simulink model "MUX_8BIT"  (R2018a)
settings: Solver=VariableStepAuto  StartTime=0.0  StopTime=10.0  RelTol=1e-3
settings Model: Creator=midog  LastModifiedBy=midog

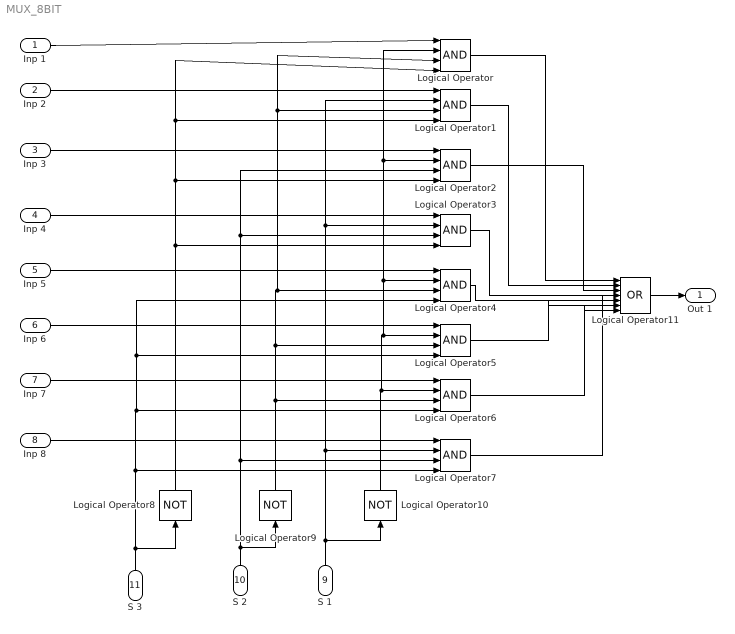
== system MUX_8BIT ==
  Inp 1 : Inport
  Inp 2 : Inport  Port=2
  Inp 3 : Inport  Port=3
  Inp 4 : Inport  Port=4
  Inp 5 : Inport  Port=5
  Inp 6 : Inport  Port=6
  Inp 7 : Inport  Port=7
  Inp 8 : Inport  Port=8
  S 1 : Inport  Port=9
  S 2 : Inport  Port=10
  S 3 : Inport  Port=11
  Logical Operator{,1..7} (8 alike) : Logic  Inputs=4  IconShape=distinctive  AllPortsSameDT=off  OutDataTypeStr=boolean
  Logical Operator10 : Logic  Operator=NOT  Inputs=4  IconShape=distinctive  AllPortsSameDT=off  OutDataTypeStr=boolean
  Logical Operator11 : Logic  Operator=OR  Inputs=8  IconShape=distinctive  AllPortsSameDT=off  OutDataTypeStr=boolean
  Logical Operator8 : Logic  Operator=NOT  Inputs=4  IconShape=distinctive  AllPortsSameDT=off  OutDataTypeStr=boolean
  Logical Operator9 : Logic  Operator=NOT  Inputs=4  IconShape=distinctive  AllPortsSameDT=off  OutDataTypeStr=boolean
  Out 1 : Outport
  wires:
  Inp 1/1 -> Logical Operator/1
  Inp 2/1 -> Logical Operator1/1
  Inp 3/1 -> Logical Operator2/1
  Inp 4/1 -> Logical Operator3/1
  Inp 5/1 -> Logical Operator4/1
  Inp 6/1 -> Logical Operator5/1
  Inp 7/1 -> Logical Operator6/1
  Inp 8/1 -> Logical Operator7/1
  S 3/1 -> Logical Operator4/4, Logical Operator5/4, Logical Operator6/4, Logical Operator7/4, Logical Operator8/1
  Logical Operator8/1 -> Logical Operator/4, Logical Operator1/4, Logical Operator2/4, Logical Operator3/4
  S 2/1 -> Logical Operator9/1, Logical Operator3/3, Logical Operator2/3, Logical Operator7/3
  Logical Operator9/1 -> Logical Operator/3, Logical Operator1/3, Logical Operator4/3, Logical Operator5/3, Logical Operator6/3
  S 1/1 -> Logical Operator10/1, Logical Operator1/2, Logical Operator3/2, Logical Operator7/2
  Logical Operator10/1 -> Logical Operator4/2, Logical Operator/2, Logical Operator2/2, Logical Operator5/2, Logical Operator6/2
  Logical Operator/1 -> Logical Operator11/1
  Logical Operator1/1 -> Logical Operator11/2
  Logical Operator2/1 -> Logical Operator11/3
  Logical Operator3/1 -> Logical Operator11/4
  Logical Operator4/1 -> Logical Operator11/5
  Logical Operator5/1 -> Logical Operator11/6
  Logical Operator6/1 -> Logical Operator11/7
  Logical Operator7/1 -> Logical Operator11/8
  Logical Operator11/1 -> Out 1/1
